simulink model "Intergration_Model_ForBasisControl"  (R2023a)
settings: Solver=ode23t  StartTime=0.0  StopTime=100  RelTol=1e-3  AbsTol=1e-3
model workspace: external: MATLAB File C:\Users\claud\OneDrive - TUM\COME -TUM\Software lab\Three_wheeled_base\simscape_1\Three_wheeled_base_DataFile1.m (data not in the file)
undefined symbols (not defined in the file or in its folder): robotData, smiData, X, Y, Z
libraries: sm_lib x202, nesl_utility x21, robotcorelib x3, fl_lib x1
(part 5 of 5)

== system Intergration_Model_ForBasisControl/Arm and Control System/Kinova Gen3 Arm/right_outer_knuckle ==
  Inertia : sm_lib/Body Elements/Inertia  InertiaType=Custom  Mass=0.00684838849401352  MassUnits=kg  CenterOfMass=[0, 0, 0]  CenterOfMassUnits=m  MomentsOfInertia=[2.70004361573169e-07, 1.38892332558312e-06, 1.26286103637978e-06]  MomentsOfInertiaUnits=kg*m^2  ProductsOfInertia=[2.82357800318817e-15, 1.56396493788199e-07, 1.59579467624491e-15]  ProductsOfInertiaUnits=kg*m^2  GraphicType=None  MarkerShape=Inertia  MarkerSize=20  GraphicVisPropType=SimpleVisualProperties  GraphicDiffuseColor=[0.5 0.5 0.5]  GraphicSpecularColor=[0.5 0.5 0.5 1.0]  GraphicAmbientColor=[0.15 0.15 0.15 1.0]  GraphicEmissiveColor=[0.0 0.0 0.0 1.0]  GraphicShininess=75  GraphicOpacity=1.0
  InertiaOriginTransform : sm_lib/Frames and Transforms/Rigid Transform  TranslationMethod=Cartesian  TranslationStandardOffset=0  TranslationStandardOffsetUnits=m  TranslationStandardAxis=+Z  TranslationCartesianOffset=[0.0178097074051638, 3.60493211424024e-11, 0.00233123458346721]  TranslationCartesianOffsetUnits=m  TranslationROffset=0  TranslationROffsetUnits=m  TranslationZOffset=0  TranslationZOffsetUnits=m  TranslationThetaOffset=0  TranslationThetaOffsetUnits=deg  RotationMethod=RotationSequence  RotationAngleUnits=deg  RotationStandardAxis=+Z  RotationAngle=0.0  RotationArbitraryAxis=[0 0 1]  FollAlignAxisA=+X  BaseAlignAxisA=+Y  FollAlignAxisB=+Y  BaseAlignAxisB=+Z  RotationSequenceAxes=BaseAxes  RotationSequence=XYZ  RotationSequenceAngles=[0, 0, 0]  RotationSequenceAnglesUnits=rad  RotationMatrix=[1 0 0; 0 1 0; 0 0 1]  Quaternion=[1 0 0 0]
  ReferenceFrame : sm_lib/Frames and Transforms/Reference Frame
  Visual : sm_lib/Body Elements/File Solid  ExtGeomFileName=Gripper85\outer_knuckle_fine.STL  UnitType=Custom  ExtGeomFileUnits=m  StepReaderType=HEX  ExportConvexHullGeometry=off  InertiaType=Custom  Mass=0  MassUnits=kg  CenterOfMass=[0, 0, 0]  CenterOfMassUnits=m  MomentsOfInertia=[0, 0, 0]  MomentsOfInertiaUnits=kg*m^2  ProductsOfInertia=[0, 0, 0]  ProductsOfInertiaUnits=kg*m^2  BasedOnType=DensityFromFile  Density=1000  DensityUnits=kg/m^3  DoExposeReferenceFrame=on  SerializedFrames=<Frames/>  GraphicType=FromGeometry  MarkerShape=Sphere  MarkerSize=10  GraphicVisPropType=SimpleVisualProperties  GraphicDiffuseColor=[0.1, 0.1, 0.1]  GraphicSpecularColor=[0.5 0.5 0.5 1.0]  GraphicAmbientColor=[0.15 0.15 0.15 1.0]  GraphicEmissiveColor=[0.0 0.0 0.0 1.0]  GraphicShininess=75  GraphicOpacity=1
  VisualOriginTransform : sm_lib/Frames and Transforms/Rigid Transform  TranslationMethod=Cartesian  TranslationStandardOffset=0  TranslationStandardOffsetUnits=m  TranslationStandardAxis=+Z  TranslationCartesianOffset=[0, 0, 0]  TranslationCartesianOffsetUnits=m  TranslationROffset=0  TranslationROffsetUnits=m  TranslationZOffset=0  TranslationZOffsetUnits=m  TranslationThetaOffset=0  TranslationThetaOffsetUnits=deg  RotationMethod=RotationSequence  RotationAngleUnits=deg  RotationStandardAxis=+Z  RotationAngle=0.0  RotationArbitraryAxis=[0 0 1]  FollAlignAxisA=+X  BaseAlignAxisA=+Y  FollAlignAxisB=+Y  BaseAlignAxisB=+Z  RotationSequenceAxes=BaseAxes  RotationSequence=XYZ  RotationSequenceAngles=[0, 0, 0]  RotationSequenceAnglesUnits=rad  RotationMatrix=[1 0 0; 0 1 0; 0 0 1]  Quaternion=[1 0 0 0]
  right_outer_finger_joint_OriginTransform : sm_lib/Frames and Transforms/Rigid Transform  TranslationMethod=Cartesian  TranslationStandardOffset=0  TranslationStandardOffsetUnits=m  TranslationStandardAxis=+Z  TranslationCartesianOffset=[0.0317095909367246, 0, -0.0016013564954687]  TranslationCartesianOffsetUnits=m  TranslationROffset=0  TranslationROffsetUnits=m  TranslationZOffset=0  TranslationZOffsetUnits=m  TranslationThetaOffset=0  TranslationThetaOffsetUnits=deg  RotationMethod=RotationSequence  RotationAngleUnits=deg  RotationStandardAxis=+Z  RotationAngle=0.0  RotationArbitraryAxis=[0 0 1]  FollAlignAxisA=+X  BaseAlignAxisA=+Y  FollAlignAxisB=+Y  BaseAlignAxisB=+Z  RotationSequenceAxes=BaseAxes  RotationSequence=XYZ  RotationSequenceAngles=[0, 0, 0]  RotationSequenceAnglesUnits=rad  RotationMatrix=[1 0 0; 0 1 0; 0 0 1]  Quaternion=[1 0 0 0]
  right_outer_knuckle_joint_AxisInvTransform : sm_lib/Frames and Transforms/Rigid Transform  TranslationMethod=Cartesian  TranslationStandardOffset=0  TranslationStandardOffsetUnits=m  TranslationStandardAxis=+Z  TranslationCartesianOffset=[0, 0, 0]  TranslationCartesianOffsetUnits=m  TranslationROffset=0  TranslationROffsetUnits=m  TranslationZOffset=0  TranslationZOffsetUnits=m  TranslationThetaOffset=0  TranslationThetaOffsetUnits=deg  RotationMethod=ArbitraryAxis  RotationAngleUnits=rad  RotationStandardAxis=+Z  RotationAngle=1.570796326794897  RotationArbitraryAxis=[-1, 0, 0]  FollAlignAxisA=+X  BaseAlignAxisA=+Y  FollAlignAxisB=+Y  BaseAlignAxisB=+Z  RotationSequenceAxes=FollowerAxes  RotationSequence=XYX  RotationSequenceAngles=[0 0 0]  RotationSequenceAnglesUnits=deg  RotationMatrix=[1 0 0; 0 1 0; 0 0 1]  Quaternion=[1 0 0 0]
  F : PMIOPort  Side=Left
  F1 : PMIOPort  Port=2  Side=Right
  connections:
  Inertia/RConn1 -- InertiaOriginTransform/RConn1
  ReferenceFrame/RConn1 -- InertiaOriginTransform/LConn1 -- right_outer_finger_joint_OriginTransform/LConn1 -- right_outer_knuckle_joint_AxisInvTransform/LConn1 -- VisualOriginTransform/LConn1
  Visual/RConn1 -- VisualOriginTransform/RConn1
  right_outer_finger_joint_OriginTransform/RConn1 -- F1/RConn1
  right_outer_knuckle_joint_AxisInvTransform/RConn1 -- F/RConn1

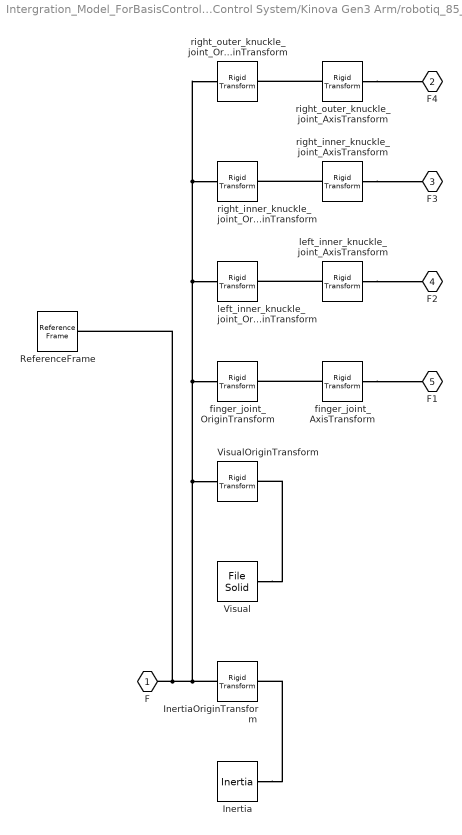
== system Intergration_Model_ForBasisControl/Arm and Control System/Kinova Gen3 Arm/robotiq_85_base_link ==
  Inertia : sm_lib/Body Elements/Inertia  InertiaType=Custom  Mass=0.30915  MassUnits=kg  CenterOfMass=[0, 0, 0]  CenterOfMassUnits=m  MomentsOfInertia=[0.00028972, 0.00030737, 0.00019914]  MomentsOfInertiaUnits=kg*m^2  ProductsOfInertia=[1.682e-12, -1.8543e-06, -5.7879e-10]  ProductsOfInertiaUnits=kg*m^2  GraphicType=None  MarkerShape=Inertia  MarkerSize=20  GraphicVisPropType=SimpleVisualProperties  GraphicDiffuseColor=[0.5 0.5 0.5]  GraphicSpecularColor=[0.5 0.5 0.5 1.0]  GraphicAmbientColor=[0.15 0.15 0.15 1.0]  GraphicEmissiveColor=[0.0 0.0 0.0 1.0]  GraphicShininess=75  GraphicOpacity=1.0
  InertiaOriginTransform : sm_lib/Frames and Transforms/Rigid Transform  TranslationMethod=Cartesian  TranslationStandardOffset=0  TranslationStandardOffsetUnits=m  TranslationStandardAxis=+Z  TranslationCartesianOffset=[0.00021987, -2.3546e-10, 0.030163]  TranslationCartesianOffsetUnits=m  TranslationROffset=0  TranslationROffsetUnits=m  TranslationZOffset=0  TranslationZOffsetUnits=m  TranslationThetaOffset=0  TranslationThetaOffsetUnits=deg  RotationMethod=RotationSequence  RotationAngleUnits=deg  RotationStandardAxis=+Z  RotationAngle=0.0  RotationArbitraryAxis=[0 0 1]  FollAlignAxisA=+X  BaseAlignAxisA=+Y  FollAlignAxisB=+Y  BaseAlignAxisB=+Z  RotationSequenceAxes=BaseAxes  RotationSequence=XYZ  RotationSequenceAngles=[0, 0, 0]  RotationSequenceAnglesUnits=rad  RotationMatrix=[1 0 0; 0 1 0; 0 0 1]  Quaternion=[1 0 0 0]
  ReferenceFrame : sm_lib/Frames and Transforms/Reference Frame
  Visual : sm_lib/Body Elements/File Solid  ExtGeomFileName=Gripper85\robotiq_85_base_link_fine.STL  UnitType=Custom  ExtGeomFileUnits=m  StepReaderType=HEX  ExportConvexHullGeometry=off  InertiaType=Custom  Mass=0  MassUnits=kg  CenterOfMass=[0, 0, 0]  CenterOfMassUnits=m  MomentsOfInertia=[0, 0, 0]  MomentsOfInertiaUnits=kg*m^2  ProductsOfInertia=[0, 0, 0]  ProductsOfInertiaUnits=kg*m^2  BasedOnType=DensityFromFile  Density=1000  DensityUnits=kg/m^3  DoExposeReferenceFrame=on  SerializedFrames=<Frames/>  GraphicType=FromGeometry  MarkerShape=Sphere  MarkerSize=10  GraphicVisPropType=SimpleVisualProperties  GraphicDiffuseColor=[0.1, 0.1, 0.1]  GraphicSpecularColor=[0.5 0.5 0.5 1.0]  GraphicAmbientColor=[0.15 0.15 0.15 1.0]  GraphicEmissiveColor=[0.0 0.0 0.0 1.0]  GraphicShininess=75  GraphicOpacity=1
  VisualOriginTransform : sm_lib/Frames and Transforms/Rigid Transform  TranslationMethod=Cartesian  TranslationStandardOffset=0  TranslationStandardOffsetUnits=m  TranslationStandardAxis=+Z  TranslationCartesianOffset=[0, 0, 0]  TranslationCartesianOffsetUnits=m  TranslationROffset=0  TranslationROffsetUnits=m  TranslationZOffset=0  TranslationZOffsetUnits=m  TranslationThetaOffset=0  TranslationThetaOffsetUnits=deg  RotationMethod=RotationSequence  RotationAngleUnits=deg  RotationStandardAxis=+Z  RotationAngle=0.0  RotationArbitraryAxis=[0 0 1]  FollAlignAxisA=+X  BaseAlignAxisA=+Y  FollAlignAxisB=+Y  BaseAlignAxisB=+Z  RotationSequenceAxes=BaseAxes  RotationSequence=XYZ  RotationSequenceAngles=[0, 0, 0]  RotationSequenceAnglesUnits=rad  RotationMatrix=[1 0 0; 0 1 0; 0 0 1]  Quaternion=[1 0 0 0]
  finger_joint_AxisTransform : sm_lib/Frames and Transforms/Rigid Transform  TranslationMethod=Cartesian  TranslationStandardOffset=0  TranslationStandardOffsetUnits=m  TranslationStandardAxis=+Z  TranslationCartesianOffset=[0, 0, 0]  TranslationCartesianOffsetUnits=m  TranslationROffset=0  TranslationROffsetUnits=m  TranslationZOffset=0  TranslationZOffsetUnits=m  TranslationThetaOffset=0  TranslationThetaOffsetUnits=deg  RotationMethod=ArbitraryAxis  RotationAngleUnits=rad  RotationStandardAxis=+Z  RotationAngle=1.570796326794897  RotationArbitraryAxis=[1, 0, 0]  FollAlignAxisA=+X  BaseAlignAxisA=+Y  FollAlignAxisB=+Y  BaseAlignAxisB=+Z  RotationSequenceAxes=FollowerAxes  RotationSequence=XYX  RotationSequenceAngles=[0 0 0]  RotationSequenceAnglesUnits=deg  RotationMatrix=[1 0 0; 0 1 0; 0 0 1]  Quaternion=[1 0 0 0]
  finger_joint_OriginTransform : sm_lib/Frames and Transforms/Rigid Transform  TranslationMethod=Cartesian  TranslationStandardOffset=0  TranslationStandardOffsetUnits=m  TranslationStandardAxis=+Z  TranslationCartesianOffset=[0.0306011444260539, 0, 0.06279201626953949]  TranslationCartesianOffsetUnits=m  TranslationROffset=0  TranslationROffsetUnits=m  TranslationZOffset=0  TranslationZOffsetUnits=m  TranslationThetaOffset=0  TranslationThetaOffsetUnits=deg  RotationMethod=RotationSequence  RotationAngleUnits=deg  RotationStandardAxis=+Z  RotationAngle=0.0  RotationArbitraryAxis=[0 0 1]  FollAlignAxisA=+X  BaseAlignAxisA=+Y  FollAlignAxisB=+Y  BaseAlignAxisB=+Z  RotationSequenceAxes=BaseAxes  RotationSequence=XYZ  RotationSequenceAngles=[0, 0, 0]  RotationSequenceAnglesUnits=rad  RotationMatrix=[1 0 0; 0 1 0; 0 0 1]  Quaternion=[1 0 0 0]
  left_inner_knuckle_joint_AxisTransform : sm_lib/Frames and Transforms/Rigid Transform  TranslationMethod=Cartesian  TranslationStandardOffset=0  TranslationStandardOffsetUnits=m  TranslationStandardAxis=+Z  TranslationCartesianOffset=[0, 0, 0]  TranslationCartesianOffsetUnits=m  TranslationROffset=0  TranslationROffsetUnits=m  TranslationZOffset=0  TranslationZOffsetUnits=m  TranslationThetaOffset=0  TranslationThetaOffsetUnits=deg  RotationMethod=ArbitraryAxis  RotationAngleUnits=rad  RotationStandardAxis=+Z  RotationAngle=1.570796326794897  RotationArbitraryAxis=[1, 0, 0]  FollAlignAxisA=+X  BaseAlignAxisA=+Y  FollAlignAxisB=+Y  BaseAlignAxisB=+Z  RotationSequenceAxes=FollowerAxes  RotationSequence=XYX  RotationSequenceAngles=[0 0 0]  RotationSequenceAnglesUnits=deg  RotationMatrix=[1 0 0; 0 1 0; 0 0 1]  Quaternion=[1 0 0 0]
  left_inner_knuckle_joint_OriginTransform : sm_lib/Frames and Transforms/Rigid Transform  TranslationMethod=Cartesian  TranslationStandardOffset=0  TranslationStandardOffsetUnits=m  TranslationStandardAxis=+Z  TranslationCartesianOffset=[0.0127000000001501, 0, 0.0693074999999639]  TranslationCartesianOffsetUnits=m  TranslationROffset=0  TranslationROffsetUnits=m  TranslationZOffset=0  TranslationZOffsetUnits=m  TranslationThetaOffset=0  TranslationThetaOffsetUnits=deg  RotationMethod=RotationSequence  RotationAngleUnits=deg  RotationStandardAxis=+Z  RotationAngle=0.0  RotationArbitraryAxis=[0 0 1]  FollAlignAxisA=+X  BaseAlignAxisA=+Y  FollAlignAxisB=+Y  BaseAlignAxisB=+Z  RotationSequenceAxes=BaseAxes  RotationSequence=XYZ  RotationSequenceAngles=[0, 0, 0]  RotationSequenceAnglesUnits=rad  RotationMatrix=[1 0 0; 0 1 0; 0 0 1]  Quaternion=[1 0 0 0]
  right_inner_knuckle_joint_AxisTransform : sm_lib/Frames and Transforms/Rigid Transform  TranslationMethod=Cartesian  TranslationStandardOffset=0  TranslationStandardOffsetUnits=m  TranslationStandardAxis=+Z  TranslationCartesianOffset=[0, 0, 0]  TranslationCartesianOffsetUnits=m  TranslationROffset=0  TranslationROffsetUnits=m  TranslationZOffset=0  TranslationZOffsetUnits=m  TranslationThetaOffset=0  TranslationThetaOffsetUnits=deg  RotationMethod=ArbitraryAxis  RotationAngleUnits=rad  RotationStandardAxis=+Z  RotationAngle=1.570796326794897  RotationArbitraryAxis=[-1, 0, 0]  FollAlignAxisA=+X  BaseAlignAxisA=+Y  FollAlignAxisB=+Y  BaseAlignAxisB=+Z  RotationSequenceAxes=FollowerAxes  RotationSequence=XYX  RotationSequenceAngles=[0 0 0]  RotationSequenceAnglesUnits=deg  RotationMatrix=[1 0 0; 0 1 0; 0 0 1]  Quaternion=[1 0 0 0]
  right_inner_knuckle_joint_OriginTransform : sm_lib/Frames and Transforms/Rigid Transform  TranslationMethod=Cartesian  TranslationStandardOffset=0  TranslationStandardOffsetUnits=m  TranslationStandardAxis=+Z  TranslationCartesianOffset=[-0.0126999999998499, 0, 0.0693075000000361]  TranslationCartesianOffsetUnits=m  TranslationROffset=0  TranslationROffsetUnits=m  TranslationZOffset=0  TranslationZOffsetUnits=m  TranslationThetaOffset=0  TranslationThetaOffsetUnits=deg  RotationMethod=RotationSequence  RotationAngleUnits=deg  RotationStandardAxis=+Z  RotationAngle=0.0  RotationArbitraryAxis=[0 0 1]  FollAlignAxisA=+X  BaseAlignAxisA=+Y  FollAlignAxisB=+Y  BaseAlignAxisB=+Z  RotationSequenceAxes=BaseAxes  RotationSequence=XYZ  RotationSequenceAngles=[0, 0, 3.14159265358979]  RotationSequenceAnglesUnits=rad  RotationMatrix=[1 0 0; 0 1 0; 0 0 1]  Quaternion=[1 0 0 0]
  right_outer_knuckle_joint_AxisTransform : sm_lib/Frames and Transforms/Rigid Transform  TranslationMethod=Cartesian  TranslationStandardOffset=0  TranslationStandardOffsetUnits=m  TranslationStandardAxis=+Z  TranslationCartesianOffset=[0, 0, 0]  TranslationCartesianOffsetUnits=m  TranslationROffset=0  TranslationROffsetUnits=m  TranslationZOffset=0  TranslationZOffsetUnits=m  TranslationThetaOffset=0  TranslationThetaOffsetUnits=deg  RotationMethod=ArbitraryAxis  RotationAngleUnits=rad  RotationStandardAxis=+Z  RotationAngle=1.570796326794897  RotationArbitraryAxis=[-1, 0, 0]  FollAlignAxisA=+X  BaseAlignAxisA=+Y  FollAlignAxisB=+Y  BaseAlignAxisB=+Z  RotationSequenceAxes=FollowerAxes  RotationSequence=XYX  RotationSequenceAngles=[0 0 0]  RotationSequenceAnglesUnits=deg  RotationMatrix=[1 0 0; 0 1 0; 0 0 1]  Quaternion=[1 0 0 0]
  right_outer_knuckle_joint_OriginTransform : sm_lib/Frames and Transforms/Rigid Transform  TranslationMethod=Cartesian  TranslationStandardOffset=0  TranslationStandardOffsetUnits=m  TranslationStandardAxis=+Z  TranslationCartesianOffset=[-0.0306011444258893, 0, 0.06279201626953949]  TranslationCartesianOffsetUnits=m  TranslationROffset=0  TranslationROffsetUnits=m  TranslationZOffset=0  TranslationZOffsetUnits=m  TranslationThetaOffset=0  TranslationThetaOffsetUnits=deg  RotationMethod=RotationSequence  RotationAngleUnits=deg  RotationStandardAxis=+Z  RotationAngle=0.0  RotationArbitraryAxis=[0 0 1]  FollAlignAxisA=+X  BaseAlignAxisA=+Y  FollAlignAxisB=+Y  BaseAlignAxisB=+Z  RotationSequenceAxes=BaseAxes  RotationSequence=XYZ  RotationSequenceAngles=[0, 0, 3.14159265358979]  RotationSequenceAnglesUnits=rad  RotationMatrix=[1 0 0; 0 1 0; 0 0 1]  Quaternion=[1 0 0 0]
  F : PMIOPort  Side=Left
  F4 : PMIOPort  Port=2  Side=Right
  F3 : PMIOPort  Port=3  Side=Right
  F2 : PMIOPort  Port=4  Side=Right
  F1 : PMIOPort  Port=5  Side=Right
  connections:
  Inertia/RConn1 -- InertiaOriginTransform/RConn1
  ReferenceFrame/RConn1 -- InertiaOriginTransform/LConn1 -- right_inner_knuckle_joint_OriginTransform/LConn1 -- right_outer_knuckle_joint_OriginTransform/LConn1 -- left_inner_knuckle_joint_OriginTransform/LConn1 -- finger_joint_OriginTransform/LConn1 -- VisualOriginTransform/LConn1 -- F/RConn1
  Visual/RConn1 -- VisualOriginTransform/RConn1
  finger_joint_AxisTransform/RConn1 -- F1/RConn1
  finger_joint_AxisTransform/LConn1 -- finger_joint_OriginTransform/RConn1
  left_inner_knuckle_joint_AxisTransform/RConn1 -- F2/RConn1
  left_inner_knuckle_joint_AxisTransform/LConn1 -- left_inner_knuckle_joint_OriginTransform/RConn1
  right_inner_knuckle_joint_AxisTransform/RConn1 -- F3/RConn1
  right_inner_knuckle_joint_AxisTransform/LConn1 -- right_inner_knuckle_joint_OriginTransform/RConn1
  right_outer_knuckle_joint_AxisTransform/RConn1 -- F4/RConn1
  right_outer_knuckle_joint_AxisTransform/LConn1 -- right_outer_knuckle_joint_OriginTransform/RConn1

== matlab function Intergration_Model_ForBasisControl/Task Scheduler ==
  settings: updateMethod=DISCRETE
  data: PlatformWaypoints1 output; PlatformWaypoints2 output; current_time input; reset_time_out_platform output; reset_time_out_arm output; arm_waypoints output; endtime_out output
function [PlatformWaypoints1,PlatformWaypoints2,reset_time_out_platform, reset_time_out_arm,arm_waypoints, endtime_out] = task_scheduler(current_time)

%-------------- Platform initialization  -----------------------------------------------------------------------
platform_destination_mat = [4000,4000;0,0;5000,0;0,0];
wheel2wheelDistance = 597;
persistent previous_platform_position previous_platform_waypoints1 previous_platform_waypoints2   
persistent reset_time_platform it_destination platform_move_begin platform_mode

if isempty(it_destination) 
    it_destination = 1;
end
if isempty(platform_move_begin) 
    
end
if isempty(platform_move_begin) 
    reset_time_platform = 0;
    platform_move_begin = 1;
    platform_mode = 0;
end
if isempty(previous_platform_waypoints1) 
    previous_platform_waypoints1 = zeros(1,2);
    previous_platform_waypoints2 = zeros(1,2);
end
if isempty(previous_platform_position)
    previous_platform_position = zeros(1,2);
end
platform_destination = zeros(1,2);
PlatformWaypoints1=previous_platform_waypoints1;
PlatformWaypoints2=previous_platform_waypoints2; 
%-------------- End of platform initialization -----------------------------------------------------------------

%-------------- Arm initialization  -------------------------------------------------------------------------
bricks_positions_mat = [0.5 ,0 , 0.05;
                        0.5 ,0.1 , 0.05];
bricks_destinations_mat = [0.5 , 0 , 0.1
                           0.5 , 0.1 , 0.1];
brick_above = [0 0 0.4];
brick_grip_pos = [0 0 0.17];
persistent it_brick  arm_mode  reset_time_arm arm_move_finished previous_Arm_Waypoints total_Arm_Waypoints end_time 
if isempty(it_brick)
    it_brick = 1 ;
end
if isempty(previous_Arm_Waypoints) 
    previous_Arm_Waypoints = zeros(8,2);
    total_Arm_Waypoints = zeros(8,9);
end
if isempty(arm_mode) 
    arm_mode = 0;
    end_time = 5;
end
if isempty(reset_time_arm) 
    reset_time_arm = 0;
end
if isempty(arm_move_finished)
    arm_move_finished = 1 ;
end
arm_waypoints = zeros(8,2);
coder.extrinsic("sm_kinovaGen3_arm_ik");
eeIgs = zeros(1,7);
%-------------- End of arm initialization -------------------------------------------------------------------

%-------------- Platform TS  -----------------------------------------------------------------------

if platform_move_begin == 1 && (arm_mode == 0 || (arm_mode == 6 && current_time - reset_time_arm > end_time + 0.1 ) || (arm_mode == 11 && current_time - reset_time_arm > end_time + 0.1 ) ) && it_destination <= size(platform_destination_mat,1)
    if arm_mode == 6
        disp("Entered platform scheduler")
    end
    platform_destination(1) = platform_destination_mat(it_destination,1);
    platform_destination(2) = platform_destination_mat(it_destination,2);
    platform_move_begin = 0;
    platform_mode = 1;
    PlatformWaypoints1(1) = previous_platform_waypoints1(2);
    PlatformWaypoints2(1) = previous_platform_waypoints2(2);
    if mod(it_destination,2) == 1
        disp("Mobile base started towards brick picking location at time: ")
        disp(current_time)
        R_map = sqrt( (platform_destination(1) - 4000)^2 + (platform_destination(2) - 0 )^2 );
        PlatformWaypoints1(2) = PlatformWaypoints1(1) +  (R_map - wheel2wheelDistance/2) * (2*pi)/4;
        PlatformWaypoints2(2) = PlatformWaypoints2(1) +  (R_map + wheel2wheelDistance/2) * (2*pi)/4;
        if (platform_destination(1) - 4000) <0
            PlatformWaypoints1(2) = - PlatformWaypoints1(2);
            PlatformWaypoints2(2) = - PlatformWaypoints2(2);
        end
    else
        disp("Mobile base started after picked brick at time: ")
        disp(current_time)
        PlatformWaypoints1(2) = PlatformWaypoints1(1) - previous_platform_waypoints1(2);
        PlatformWaypoints2(2) = PlatformWaypoints2(1) - previous_platform_waypoints2(2);
    end  
    previous_platform_waypoints1 = PlatformWaypoints1;
    previous_platform_waypoints2 = PlatformWaypoints2;
    reset_time_platform = current_time;
    previous_platform_position = platform_destination;
    if size(platform_destination_mat,1) >= it_destination
        it_destination = it_destination + 1;
    end
end
PlatformWaypoints2 = - PlatformWaypoints2 / 80;
PlatformWaypoints1 =  PlatformWaypoints1 / 80;
reset_time_out_platform = reset_time_platform;


if (platform_mode == 1) && (current_time - reset_time_platform >= 7 + 0.2)   % Waypoints end time is [3,1,3]--> 3 + 1 + 3 == 7
    disp("Mobile base movement finished at time")
    disp(current_time)
    platform_mode = 0 ;
    if arm_mode == 0 || arm_mode == 11
        arm_mode = 1 ;
    elseif arm_mode == 6
        arm_mode = 7 ;
    end        

end
%-------------- End of platform TS  -----------------------------------------------------------------------

%-------------- Arm TS  -----------------------------------------------------------------------
if arm_mode == 1
    arm_mode = 2 ;
    disp("Arm started approaching to pick at time")
    disp(current_time)
    brick_pick_pos = bricks_positions_mat(it_brick,:);
    brick_place_pos = bricks_destinations_mat(it_brick,:);
    TR_frame = [
    [brick_pick_pos+brick_above,[180 0 0]];...
    [brick_pick_pos+brick_grip_pos,[180 0 0]];...
    [brick_pick_pos+brick_grip_pos,[180 0 0]];...
    [brick_pick_pos+brick_above,[180 0 0]];...
    [brick_place_pos+brick_grip_pos,[180 0 0]];...
    [brick_place_pos+brick_grip_pos,[180 0 0]];...
    [brick_place_pos+brick_above,[180 0 0]]];
    [solution,solvedFlag] =  sm_kinovaGen3_arm_ik(TR_frame,eeIgs);

    total_Arm_Waypoints(1:7,2:size(TR_frame,1)+1) = solution;
    total_Arm_Waypoints(1:7,2:size(TR_frame,1)+1) = total_Arm_Waypoints(1:7,2:size(TR_frame,1)+1)./180*pi;
    total_Arm_Waypoints(:,1) = 0;
    total_Arm_Waypoints(:,size(TR_frame,1)+2) = 0;
    total_Arm_Waypoints(8,:)=0;
    total_Arm_Waypoints(8,4:6)=0.5;
    total_Arm_Waypoints(8,7)=-0.5;
    
    arm_waypoints(:,2) = total_Arm_Waypoints(:,2);
    previous_Arm_Waypoints = arm_waypoints;
    reset_time_arm = current_time ;
    end_time = 5;
elseif arm_mode == 2 && current_time - reset_time_arm > end_time + 0.1
    disp("Arm started going down to pick at time")
    disp(current_time)
    arm_mode = 3;
    arm_waypoints(:,1) = total_Arm_Waypoints(:,2);
    arm_waypoints(:,2) = total_Arm_Waypoints(:,3);
    previous_Arm_Waypoints = arm_waypoints;
    reset_time_arm = current_time ;
    end_time = 1;
elseif arm_mode == 3 && current_time - reset_time_arm > end_time + 0.1
    disp("Arm closed grip to pick at time")
    disp(current_time)
    arm_mode = 4;
    arm_waypoints(:,1) = total_Arm_Waypoints(:,3);
    arm_waypoints(:,2) = total_Arm_Waypoints(:,4);
    previous_Arm_Waypoints = arm_waypoints;
    reset_time_arm = current_time ;
    end_time = 1;
elseif arm_mode == 4 && current_time - reset_time_arm > end_time + 0.1
    disp("Arm picked and the gripper moved a bit higher")
    disp(current_time)
    arm_mode = 5;
    arm_waypoints(:,1) = total_Arm_Waypoints(:,4);
    arm_waypoints(:,2) = total_Arm_Waypoints(:,5); %% This might need modification
    previous_Arm_Waypoints = arm_waypoints;
    reset_time_arm = current_time ;
    end_time = 1;
elseif arm_mode == 5 && current_time - reset_time_arm > end_time + 0.1
    disp("Arm moved to highest position")
    disp(current_time)
    arm_mode = 6;
    platform_move_begin = 1;
    arm_waypoints(:,1) = total_Arm_Waypoints(:,5);
    arm_waypoints(1:7,2) = zeros(7,1); %% This might need modification
    arm_waypoints(8,2) = 0.5;
    previous_Arm_Waypoints = arm_waypoints;
    reset_time_arm = current_time ;
    end_time = 5;
elseif arm_mode == 7 && current_time  - reset_time_arm > end_time + 0.1
     disp("Arm started approaching to place the brick at time")
     disp(current_time)
     arm_mode = 8;
     arm_waypoints(1:7,1) = zeros(7,1); %% This might need modification
     arm_waypoints(8,1) = 0.5;
     arm_waypoints(:,2) = total_Arm_Waypoints(:,6); %% This might need modification
     previous_Arm_Waypoints = arm_waypoints;
     reset_time_arm = current_time ;
     end_time = 7;
 elseif arm_mode == 8 && current_time - reset_time_arm > end_time + 0.1
     disp("Arm opened grips")
     disp(current_time)
     arm_mode = 9;
     arm_waypoints(:,1) = total_Arm_Waypoints(:,6); %% This might need modification
     arm_waypoints(:,2) = total_Arm_Waypoints(:,7); %% This might need modification
     previous_Arm_Waypoints = arm_waypoints;
     reset_time_arm = current_time ;
     end_time = 1;
  elseif arm_mode == 9 && current_time - reset_time_arm > end_time + 0.1
     disp("Arm went upper after it left the brick")
     disp(current_time)
     arm_mode = 10;
     arm_waypoints(:,1) = total_Arm_Waypoints(:,7); %% This might need modification
     arm_waypoints(:,2) = total_Arm_Waypoints(:,8); %% This might need modification
     previous_Arm_Waypoints = arm_waypoints;
     reset_time_arm = current_time ;
     end_time = 1;
  elseif arm_mode == 10 && current_time - reset_time_arm > end_time + 0.1
     disp("Arm went initial position")
     disp(current_time)
     platform_move_begin = 1;
     arm_mode = 11;
     arm_waypoints(:,1) = total_Arm_Waypoints(:,8); %% This might need modification
     arm_waypoints(:,2) = zeros(8,1); %% This might need modification
     previous_Arm_Waypoints = arm_waypoints;
     reset_time_arm = current_time ;
     end_time = 5;
     it_brick = it_brick + 1;
end

reset_time_out_arm = reset_time_arm ;
arm_waypoints = previous_Arm_Waypoints;
endtime_out = end_time;
%-------------- End of TS  --------------------------------------------------------------------

end
